simulink subsystem "CAVsSensorFusion"  (R2022b)
settings: Solver=VariableStepAuto  StartTime=0.0  StopTime=10.0  RelTol=1e-3
settings Model: DefaultTestHarness=CAVsSensorFusion_Harness1  Creator=smryk  LastModifiedBy=lupas

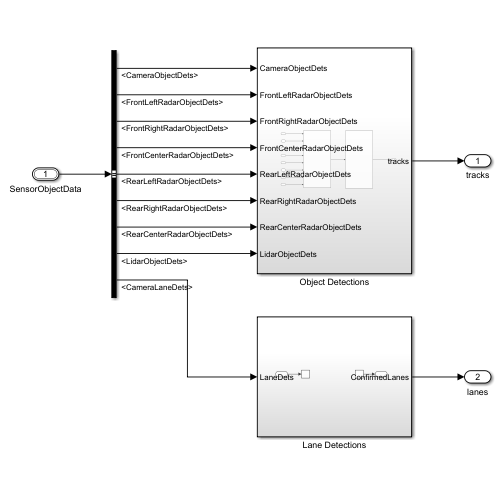
[thumbnail: Simulink's stored preview of the top-level diagram]
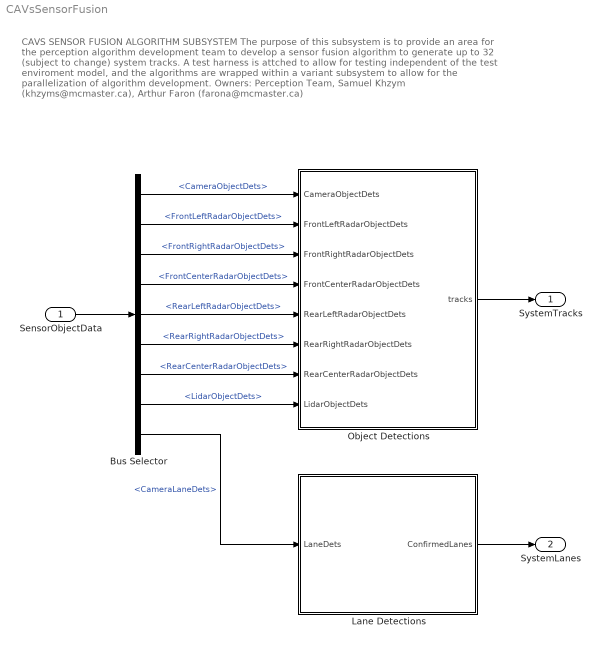
== system CAVsSensorFusion ==
  note: CAVS SENSOR FUSION ALGORITHM SUBSYSTEM
      |
      | The purpose of this subsystem is to provide an area for the perception algorithm development team to develop a sensor fusion algorithm to generate up to 32 (subject to change) system tracks. A test harness is attched to allow for testing independent of the test enviroment model, and the algorithms are wrapped within a variant subsystem to allow for the parallelization of algorithm development.
      |
      | Owners: Perception Team, Samuel Khzym (khzyms@mcmaster.ca), Arthur Faron (farona@mcmaster.ca)
  SensorObjectData : Inport  OutDataTypeStr=Bus: SensorObjectData
  Bus Selector : BusSelector  OutputSignals=CameraObjectDets,FrontLeftRadarObjectDets,FrontRightRadarObjectDets,FrontCenterRadarObjectDets,RearLeftRadarObjectDets,RearRightRadarObjectDets,RearCenterRadarObjectDets,LidarObjectDets,CameraLaneDets
  Lane Detections : Subsystem
  Object Detections : Subsystem
  SystemTracks : Outport  OutDataTypeStr=Bus: SystemTracks
  SystemLanes : Outport  Port=2
  wires:
  SensorObjectData/1 -> Bus Selector/1
  Bus Selector/9 -> Lane Detections/1(LaneDets)  "<CameraLaneDets>"
  Bus Selector/1 -> Object Detections/1(CameraObjectDets)  "<CameraObjectDets>"
  Bus Selector/2 -> Object Detections/2(FrontLeftRadarObjectDets)  "<FrontLeftRadarObjectDets>"
  Bus Selector/3 -> Object Detections/3(FrontRightRadarObjectDets)  "<FrontRightRadarObjectDets>"
  Bus Selector/4 -> Object Detections/4(FrontCenterRadarObjectDets)  "<FrontCenterRadarObjectDets>"
  Bus Selector/5 -> Object Detections/5(RearLeftRadarObjectDets)  "<RearLeftRadarObjectDets>"
  Bus Selector/6 -> Object Detections/6(RearRightRadarObjectDets)  "<RearRightRadarObjectDets>"
  Bus Selector/7 -> Object Detections/7(RearCenterRadarObjectDets)  "<RearCenterRadarObjectDets>"
  Bus Selector/8 -> Object Detections/8(LidarObjectDets)  "<LidarObjectDets>"
  Object Detections/1(tracks) -> SystemTracks/1
  Lane Detections/1(ConfirmedLanes) -> SystemLanes/1

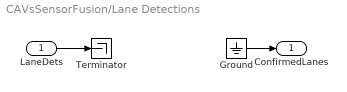
== system CAVsSensorFusion/Lane Detections ==
  LaneDets : Inport
  Ground : Ground
  Terminator : Terminator
  ConfirmedLanes : Outport
  wires:
  LaneDets/1 -> Terminator/1
  Ground/1 -> ConfirmedLanes/1

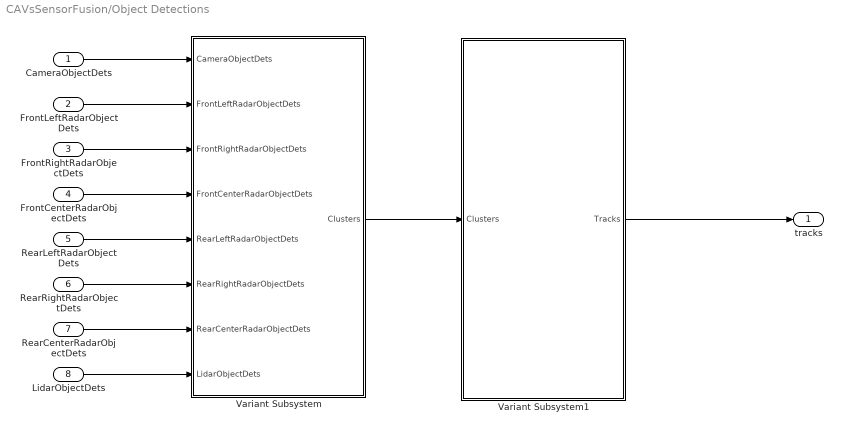
== system CAVsSensorFusion/Object Detections ==
  CameraObjectDets : Inport
  FrontLeftRadarObjectDets : Inport  Port=2
  FrontRightRadarObjectDets : Inport  Port=3
  FrontCenterRadarObjectDets : Inport  Port=4
  RearLeftRadarObjectDets : Inport  Port=5
  RearRightRadarObjectDets : Inport  Port=6
  RearCenterRadarObjectDets : Inport  Port=7
  LidarObjectDets : Inport  Port=8
  Variant Subsystem : Subsystem  Variant=on
  Variant Subsystem1 : Subsystem  Variant=on
  tracks : Outport
  wires:
  CameraObjectDets/1 -> Variant Subsystem/1(CameraObjectDets)
  FrontLeftRadarObjectDets/1 -> Variant Subsystem/2(FrontLeftRadarObjectDets)
  FrontRightRadarObjectDets/1 -> Variant Subsystem/3(FrontRightRadarObjectDets)
  FrontCenterRadarObjectDets/1 -> Variant Subsystem/4(FrontCenterRadarObjectDets)
  RearLeftRadarObjectDets/1 -> Variant Subsystem/5(RearLeftRadarObjectDets)
  RearRightRadarObjectDets/1 -> Variant Subsystem/6(RearRightRadarObjectDets)
  RearCenterRadarObjectDets/1 -> Variant Subsystem/7(RearCenterRadarObjectDets)
  LidarObjectDets/1 -> Variant Subsystem/8(LidarObjectDets)
  Variant Subsystem/1(Clusters) -> Variant Subsystem1/1(Clusters)
  Variant Subsystem1/1(Tracks) -> tracks/1

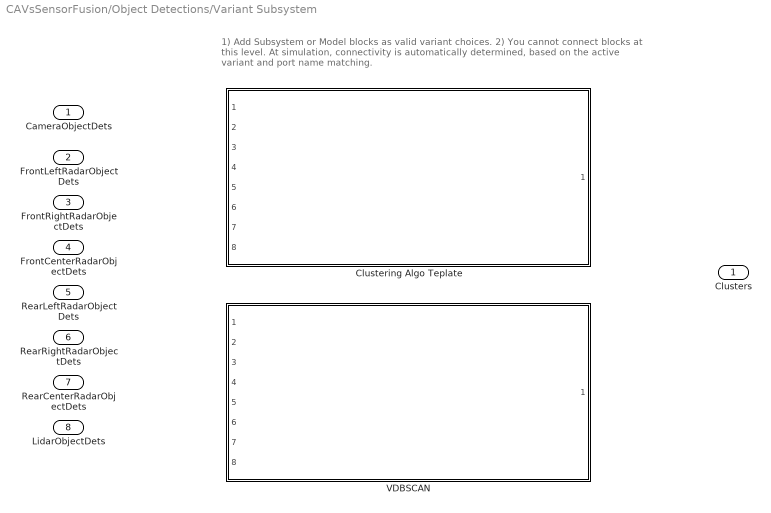
== system CAVsSensorFusion/Object Detections/Variant Subsystem ==
  note: 1) Add Subsystem or Model blocks as valid variant choices.
      | 2) You cannot connect blocks at this level. At simulation, connectivity is automatically
      | determined, based on the active variant and port name matching.
  CameraObjectDets : Inport
  FrontLeftRadarObjectDets : Inport  Port=2
  FrontRightRadarObjectDets : Inport  Port=3
  FrontCenterRadarObjectDets : Inport  Port=4
  RearLeftRadarObjectDets : Inport  Port=5
  RearRightRadarObjectDets : Inport  Port=6
  RearCenterRadarObjectDets : Inport  Port=7
  LidarObjectDets : Inport  Port=8
  Clustering Algo Teplate : Subsystem  ReferencedSubsystem=ClusteringAlgoTemplate
  VDBSCAN : Subsystem  VariantControl=(default)  ReferencedSubsystem=ClusteringAlgoTemplate
  Clusters : Outport  OutDataTypeStr=Bus: BusObjectDetections1

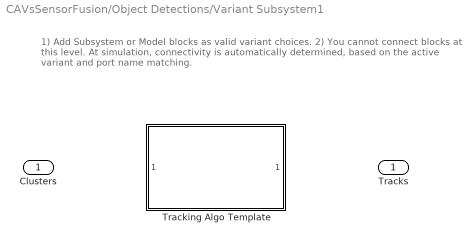
== system CAVsSensorFusion/Object Detections/Variant Subsystem1 ==
  note: 1) Add Subsystem or Model blocks as valid variant choices.
      | 2) You cannot connect blocks at this level. At simulation, connectivity is automatically
      | determined, based on the active variant and port name matching.
  Clusters : Inport  OutDataTypeStr=Bus: BusObjectDetections1
  Tracking Algo Template : Subsystem  VariantControl=(default)  ReferencedSubsystem=TrackingAlgoTemplate
  Tracks : Outport  OutDataTypeStr=Bus: SystemTracks
